simulink model "Fahrdynamikregelung"  (R2022b)
settings: Solver=ode1  StartTime=0.0  StopTime=10.0  FixedStep=Ts  RelTol=1e-3
InitFcn:
  | run("Fzg_Par.m")
values from neighbouring files (symbols this model uses):
  aero_balance_rear = 55/100    (= 0.55)    [Fzg_Par.m]    (also in Fzg_par.m)
  c_alpha_H = 13400    [Fzg_Par.m]    (also in Fzg_par.m)
  c_alpha_V = 9300    [Fzg_Par.m]    (also in Fzg_par.m)
  c_DA = 3.9    [Fzg_Par.m]    (also in Fzg_par.m)
  Dyn_Reifenradius = 0.23    [Fzg_Par.m]    (also in Fzg_par.m)
  h_COG = 300/1000    (= 0.3)    [Fzg_Par.m]    (also in Fzg_par.m)
  J_Rad = 0.2656    [Fzg_Par.m]
  K_PD = 5    [Fzg_Par.m]
  K_T = 0.62    [Fzg_Par.m]
  L001_APPS1 = [7.99989318848 7.99989318848 7.99989318848 7.99989318848 7.99989318848 7.99989318848 7.99989318848 7.99989318848 7.99989318848 7.99989318848 7.99989318848 7.99989318848 ... (3961 elements, 3961x1)]    [TestData24.mat]
  L001_GPSSpeed = [0.148407205939 0.148407205939 0.148407205939 0.148407205939 0.148407205939 0.148407205939 0.148407205939 0.148407205939 0.148407205939 0.148407205939 0.153283953667 0.202051386237 ... (3961 elements, 3961x1)]    [TestData24.mat]
  L001_InlineAcc = [-0.0102365128696 -0.0101919434965 -0.00925597175956 -0.0068023907952 -0.00259832036681 0.00465657003224 0.0166592858732 0.0341619476676 0.0555711686611 0.0739719197154 0.0942579805851 0.102946907282 ... (3961 elements, 3961x1)]    [TestData24.mat]
  L001_INVRERPM = [228.575454712 228.575454712 228.575454712 228.575454712 228.575454712 228.575454712 228.575454712 228.575454712 228.575454712 228.575454712 229.405059814 237.701187134 ... (3961 elements, 3961x1)]    [TestData24.mat]
  L001_LateralAcc = [-0.171782910824 -0.171881780028 -0.171881780028 -0.171881780028 -0.17187024653 -0.171626374125 -0.171095818281 -0.169845193624 -0.168227121234 -0.169884741306 -0.173443824053 -0.169364064932 ... (3961 elements, 3961x1)]    [TestData24.mat]
  L001_Steeringangle = [-0.000259418739006 -0.000259418739006 -0.000259418739006 -0.000259418739006 -0.000259418739006 -0.000259418739006 -0.000259418739006 -0.000259418739006 -0.000259418739006 -0.000259418739006 -0.000259418739006 -0.000259418739006 ... (3961 elements, 3961x1)]    [TestData24.mat]
  L001_time = [0 0.019999999553 0.0399999991059 0.0599999986589 0.0799999982119 0.10000000149 0.119999997318 0.140000000596 0.159999996424 0.180000007153 0.20000000298 0.219999998808 ... (3961 elements, 3961x1)]    [TestData24.mat]
  L001_YawRate = [0.023690149188 0.0136420829222 0.00359401665628 -0.0035233637318 -0.0120642203838 -0.0241218991578 -0.0424596183002 -0.0578666552901 -0.0431294925511 0.0049337586388 0.0141444858164 -0.0101383412257 ... (3961 elements, 3961x1)]    [TestData24.mat]
  L038_ACcurrentINVL = [99.4390869141 109.504394531 119.569709778 129.252166748 135.488876343 141.725585938 147.962295532 154.199005127 160.137954712 163.397140503 166.656311035 169.915481567 ... (1550 elements, 1550x1)]    [Lap38Data.mat]
  L038_ACcurrentINVR = [20.6730155945 25.7066345215 30.7402534485 36.3266334534 46.8878517151 57.4490699768 68.0102920532 78.5715103149 88.6779708862 94.6916427612 100.705307007 106.718971252 ... (1550 elements, 1550x1)]    [Lap38Data.mat]
  L038_DCcurrentINVL = [23.7739772797 26.0139312744 28.2538833618 30.4728279114 32.5027122498 34.5325965881 36.5624809265 38.5923652649 40.5376625061 41.7216491699 42.9056396484 44.089630127 ... (1550 elements, 1550x1)]    [Lap38Data.mat]
  L038_DCcurrentINVR = [4.40954971313 5.53267717361 6.65580463409 7.92606782913 10.5205507278 13.1150331497 15.7095165253 18.3039989471 20.8878383636 23.3758850098 25.8639297485 28.3519744873 ... (1550 elements, 1550x1)]    [Lap38Data.mat]
  L038_time = [0 0.019999999553 0.0399999991059 0.0599999986589 0.0799999982119 0.10000000149 0.119999997318 0.140000000596 0.159999996424 0.180000007153 0.20000000298 0.219999998808 ... (1550 elements, 1550x1)]    [Lap38Data.mat]    (also in Testrunde_PATZE.mat)
  L038_VTS = [491.347839355 491.925415039 492.502990723 492.660247803 489.034515381 485.408782959 481.783050537 478.157287598 474.759063721 473.408447266 472.057830811 470.707214355 ... (1550 elements, 1550x1)]    [Lap38Data.mat]
  l_fzg = 1300/1000    (= 1.3)    [Fzg_Par.m]    (also in Fzg_par.m)
  l_H_fzg = 507/1000    (= 0.507)    [Fzg_Par.m]    (also in Fzg_par.m)
  l_V_fzg = 1023/1000    (= 1.023)    [Fzg_Par.m]    (also in Fzg_par.m)
  m_Front = m_fzg * 0.4    (= 129.4)    [Fzg_Par.m]    (also in Fzg_par.m)
  m_fzg = 241.5 + 82    (= 323.5)    [Fzg_Par.m]    (also in Fzg_par.m)
  m_Rear = m_fzg - m_Front    (= 194.1)    [Fzg_Par.m]    (also in Fzg_par.m)
  ss_A = [-(c_alpha_V*l_V_fzg^2+c_alpha_H*l_H_fzg^2)/(J_fzg_z*v_x) (c_alpha_H*l_H_fzg-c_alpha_V*l_V_fzg)/J_fzg_z ... (first row only)    [Fzg_Par.m]    (also in Fzg_par.m)
  ss_B = [(c_alpha_V*l_V_fzg)/J_fzg_z -(c_alpha_H*l_H_fzg)/J_fzg_z ... (first row only)    [Fzg_Par.m]    (also in Fzg_par.m)
  ss_C = [1 0]    [Fzg_Par.m]    (also in Fzg_par.m)
  ss_D = [0 0]    [Fzg_Par.m]    (also in Fzg_par.m)
  t_H_fzg = 1200/1000    (= 1.2)    [Fzg_Par.m]    (also in Fzg_par.m)
  T_p = T_v/10    (= 0.01)    [Fzg_Par.m]
  T_v = 0.1    [Fzg_Par.m]
libraries: simulink x2
settings Model: Creator=timos  LastModifiedBy=timos

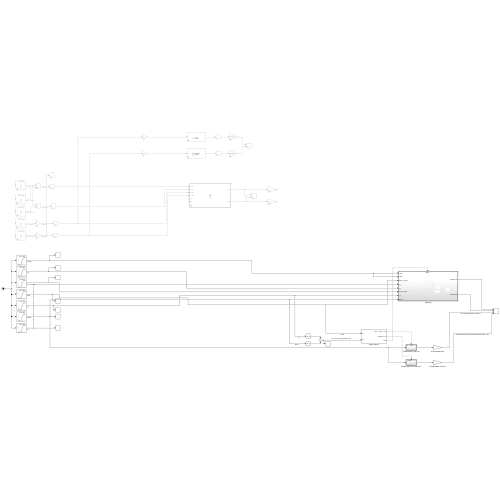
[thumbnail: Simulink's stored preview of the top-level diagram]
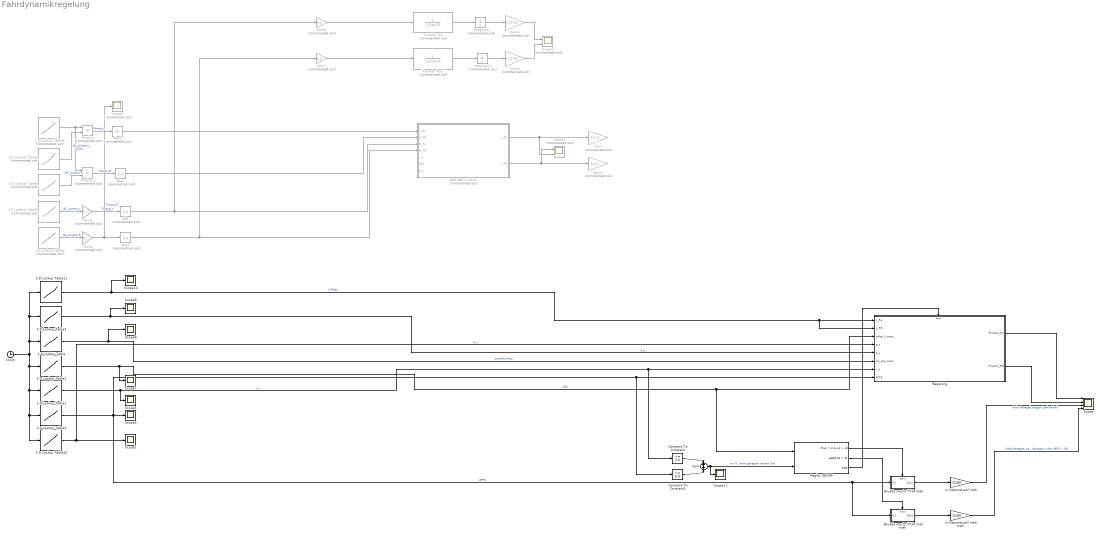
== system Fahrdynamikregelung ==
  1-D Lookup Table : Lookup_n-D  NumberOfTableDimensions=1  BreakpointsForDimension1=L001_time  Table=L001_YawRate  InternalRulePriority=Speed  RndMeth=Simplest
  1-D Lookup Table1 : Lookup_n-D  NumberOfTableDimensions=1  BreakpointsForDimension1=L001_time  Table=L001_GPSSpeed/3.6  InternalRulePriority=Speed  RndMeth=Simplest
  1-D Lookup Table10 : Lookup_n-D  NumberOfTableDimensions=1  BreakpointsForDimension1=L001_time  Table=L001_InlineAcc*9.81  InternalRulePriority=Speed  RndMeth=Simplest
  1-D Lookup Table11 : Lookup_n-D  NumberOfTableDimensions=1  BreakpointsForDimension1=L001_time  Table=L001_INVRERPM/(10*60*4.3)  InternalRulePriority=Speed  RndMeth=Simplest
  1-D Lookup Table2 : Lookup_n-D  NumberOfTableDimensions=1  BreakpointsForDimension1=L001_time  Table=L001_Steeringangle*0.36  InternalRulePriority=Speed  RndMeth=Simplest
  1-D Lookup Table3 : Lookup_n-D  NumberOfTableDimensions=1  BreakpointsForDimension1=L001_time  Table=L001_LateralAcc*9.81  InternalRulePriority=Speed  RndMeth=Simplest
  1-D Lookup Table4 : Lookup_n-D  NumberOfTableDimensions=1  BreakpointsForDimension1=L001_time  Table=L001_APPS1  InternalRulePriority=Speed  RndMeth=Simplest
  1-D Lookup Table5 : Lookup_n-D  Commented=on  NumberOfTableDimensions=1  BreakpointsForDimension1=L038_time  Table=L038_DCcurrentINVL  InternalRulePriority=Speed  RndMeth=Simplest
  1-D Lookup Table6 : Lookup_n-D  Commented=on  NumberOfTableDimensions=1  BreakpointsForDimension1=L038_time  Table=L038_DCcurrentINVR  InternalRulePriority=Speed  RndMeth=Simplest
  1-D Lookup Table7 : Lookup_n-D  Commented=on  NumberOfTableDimensions=1  BreakpointsForDimension1=L038_time  Table=L038_ACcurrentINVL  InternalRulePriority=Speed  RndMeth=Simplest
  1-D Lookup Table8 : Lookup_n-D  Commented=on  NumberOfTableDimensions=1  BreakpointsForDimension1=L038_time  Table=L038_ACcurrentINVR  InternalRulePriority=Speed  RndMeth=Simplest
  1-D Lookup Table9 : Lookup_n-D  Commented=on  NumberOfTableDimensions=1  BreakpointsForDimension1=L038_time  Table=L038_VTS  InternalRulePriority=Speed  RndMeth=Simplest
  Abs{,1..3} (4 alike) : Abs  Commented=on  SaturateOnIntegerOverflow=off
  Brudda macht TY24 meh : Subsystem  TreatAsAtomicUnit=on
  Brudda macht TY24 meh meh : Subsystem  TreatAsAtomicUnit=on
  Clock : Clock
  Compare To Constant : simulink/Logic and Bit Operations/Compare To Constant  relop=<=  const=2.0  OutDataTypeStr=boolean
  Compare To Constant1 : simulink/Logic and Bit Operations/Compare To Constant  relop=<=  const=5.0  OutDataTypeStr=boolean
  Gain : Gain  Commented=on  Gain=1/4.3
  Gain1 : Gain  Commented=on  Gain=K_T
  Gain2 : Gain  Commented=on  Gain=K_T
  Gain3 : Gain  Commented=on  Gain=1/4.3
  Gain4 : Gain  Commented=on  Gain=1/(2*pi)
  Gain5 : Gain  Commented=on  Gain=1/(2*pi)
  Gain6 : Gain  Commented=on  Gain=4.3
  Gain7 : Gain  Commented=on  Gain=4.3
  Integrator : Integrator  Commented=on
  Integrator1 : Integrator  Commented=on
  MATLAB Function : MATLAB Function  Commented=on  TreatAsAtomicUnit=on
  Product : Product  Commented=on
  Product1 : Product  Commented=on
  Regelung : Subsystem
  Regler ON/OFF : If  NumInputs=2  IfExpression=u1 < 3 & u1 > -3  ElseIfExpressions=u2 > 0
  Scope : Scope  NumInputPorts=4
  Scope{1,4..5,7..11} (8 alike) : Scope
  Scope2 : Scope  Commented=on  NumInputPorts=2
  Scope3 : Scope  Commented=on  NumInputPorts=2
  Scope6 : Scope  Commented=on
  Sum : Sum  Inputs=+|+  OutDataTypeStr=double
  Transfer Fcn : TransferFcn  Commented=on  Denominator=[J_Rad 0]
  Transfer Fcn1 : TransferFcn  Commented=on  Denominator=[J_Rad 0]
  in Dezimalzahl meh : Gain  Gain=1/100
  in Dezimalzahl meh meh : Gain  Gain=1/100
  wires:
  Clock/1 -> 1-D Lookup Table/1, 1-D Lookup Table11/1, 1-D Lookup Table3/1, 1-D Lookup Table2/1, 1-D Lookup Table10/1, 1-D Lookup Table4/1, 1-D Lookup Table1/1
  1-D Lookup Table3/1 -> Scope9/1, Regelung/5(a_y)  "a_y"
  1-D Lookup Table5/1 -> Product/2  "DC_current_L"
  1-D Lookup Table7/1 -> Gain2/1  "AC_current_L"
  1-D Lookup Table8/1 -> Gain1/1  "AC_current_R"
  Gain2/1 -> Abs/1  "Torque_L"
  Gain1/1 -> Abs1/1, Scope6/1  "Torque_R"
  1-D Lookup Table9/1 -> Product1/1, Product/1  "V_TS"
  1-D Lookup Table6/1 -> Product1/2  "DC_current_R"
  Product/1 -> Abs3/1  "Power_L"
  Product1/1 -> Abs2/1  "Power_R"
  Abs/1 -> Gain6/1, MATLAB Function/3(M_RL)
  Abs1/1 -> Gain7/1, MATLAB Function/4(M_RR)
  Abs2/1 -> MATLAB Function/2(P_RR)
  Abs3/1 -> MATLAB Function/1(P_RL)
  MATLAB Function/1(n_RL) -> Scope2/2, Gain/1
  MATLAB Function/2(n_RR) -> Scope2/1, Gain3/1
  1-D Lookup Table/1 -> Scope8/1, Regelung/6(psi_dot_mess)  "psi_dot_mess"
  1-D Lookup Table4/1 -> Regelung/8(APPS), Compare To Constant1/1, Scope4/1, Brudda macht TY24 meh meh/1(In1), Brudda macht TY24 meh/1(In1)  "APPS"
  1-D Lookup Table1/1 -> Scope5/1, Regelung/7(v_x), Compare To Constant/1  "v_x"
  1-D Lookup Table2/1 -> Scope7/1, Regler ON/OFF/1, Regelung/3("delta_V_mess ")  "SAS"
  1-D Lookup Table10/1 -> Scope1/1, Regelung/4(a_x)  "a_x"
  Regelung/2(Produkt_RR) -> Scope/2
  Regelung/1(Produkt_RL) -> Scope/1
  Brudda macht TY24 meh/1(Out1) -> in Dezimalzahl meh/1
  Transfer Fcn1/1 -> Integrator1/1
  Transfer Fcn/1 -> Integrator/1
  Integrator1/1 -> Gain5/1
  Integrator/1 -> Gain4/1
  Gain4/1 -> Scope3/1
  Gain5/1 -> Scope3/2
  Gain7/1 -> Transfer Fcn1/1
  Gain6/1 -> Transfer Fcn/1
  1-D Lookup Table11/1 -> Scope10/1, Regelung/2(n_RR), Regelung/1(n_RL)  "n_Rear"
  in Dezimalzahl meh/1 -> Scope/3  "Nicht Geregelt wegen Lenkwinkel"
  in Dezimalzahl meh meh/1 -> Scope/4  "Nicht Geregelt wegen Arschlangsam oder APPS < 5%"
  Brudda macht TY24 meh meh/1(Out1) -> in Dezimalzahl meh meh/1
  Regler ON/OFF/1 -> Brudda macht TY24 meh/Action
  Regler ON/OFF/2 -> Brudda macht TY24 meh meh/Action
  Regler ON/OFF/3 -> Regelung/Action
  Compare To Constant/1 -> Sum/1
  Compare To Constant1/1 -> Sum/2
  Sum/1 -> Scope11/1, Regler ON/OFF/2  "nur 0, wenn geregelt werden Soll"

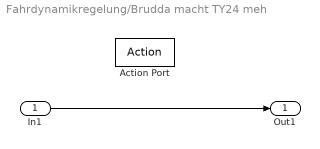
== system Fahrdynamikregelung/Brudda macht TY24 meh ==
  In1 : Inport
  Action Port : ActionPort  ActionPortLabel=if(u1 < 3 & u1 > -3)
  Out1 : Outport
  wires:
  In1/1 -> Out1/1

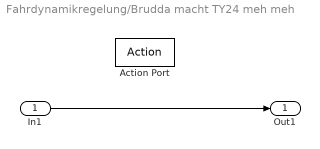
== system Fahrdynamikregelung/Brudda macht TY24 meh meh ==
  In1 : Inport
  Action Port : ActionPort  ActionPortLabel=elseif(u2 > 0)
  Out1 : Outport
  wires:
  In1/1 -> Out1/1

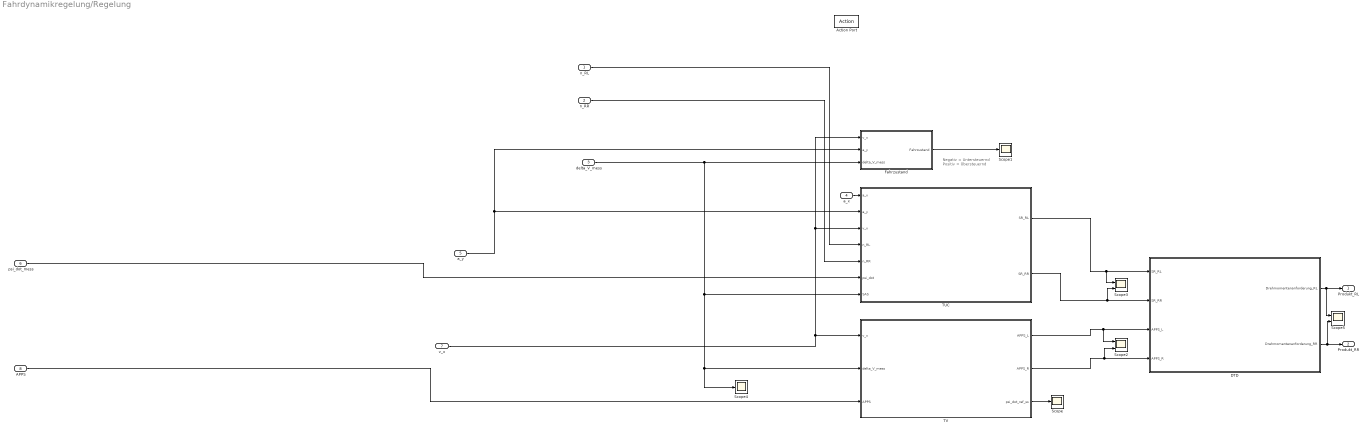
== system Fahrdynamikregelung/Regelung ==
  note: Negativ = Untersteuernd
      | Positiv = Übersteuernd
  n_RL : Inport
  n_RR : Inport  Port=2
  "delta_V_mess " : Inport  Port=3
  a_x : Inport  Port=4
  a_y : Inport  Port=5
  psi_dot_mess : Inport  Port=6
  v_x : Inport  Port=7
  APPS : Inport  Port=8
  Action Port : ActionPort  ActionPortLabel=else
  DTD : Subsystem
  Fahrzustand : Subsystem
  Scope : Scope
  Scope1 : Scope
  Scope2 : Scope  NumInputPorts=2
  Scope3 : Scope  NumInputPorts=2
  Scope4 : Scope
  Scope5 : Scope  NumInputPorts=2
  TUC : Subsystem
  TV : Subsystem
  Produkt_RL : Outport
  Produkt_RR : Outport  Port=2
  wires:
  v_x/1 -> Fahrzustand/1(v_x), TUC/3(v_x), TV/1(v_x)
  a_y/1 -> TUC/2(a_y), Fahrzustand/2(a_y)
  n_RR/1 -> TUC/5(n_RR)
  TUC/1(SR_RL) -> Scope3/1, DTD/1(SR_RL)
  TUC/2(SR_RR) -> Scope3/2, DTD/2(SR_RR)
  Fahrzustand/1(Fahrzustand) -> Scope1/1
  TV/1(APPS_L) -> Scope2/1, DTD/3(APPS_L)
  TV/3(psi_dot_ref_ss) -> Scope/1
  TV/2(APPS_R) -> Scope2/2, DTD/4(APPS_R)
  psi_dot_mess/1 -> TUC/6(psi_dot)
  n_RL/1 -> TUC/4(n_RL)
  APPS/1 -> TV/3(APPS)
  a_x/1 -> TUC/1(a_x)
  "delta_V_mess "/1 -> TV/2(delta_V_mess), Scope4/1, TUC/7(SAS), Fahrzustand/3("delta_V_mess ")
  DTD/1(Drehmomentenanforderung_RL) -> Scope5/1, Produkt_RL/1
  DTD/2(Drehmomentenanforderung_RR) -> Scope5/2, Produkt_RR/1

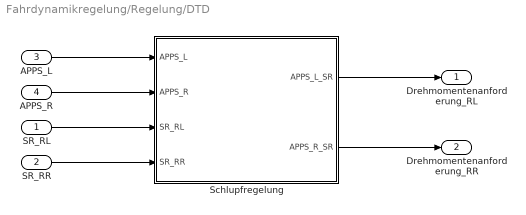
== system Fahrdynamikregelung/Regelung/DTD ==
  SR_RL : Inport
  SR_RR : Inport  Port=2
  APPS_L : Inport  Port=3
  APPS_R : Inport  Port=4
  Schlupfregelung : MATLAB Function  TreatAsAtomicUnit=on
  Drehmomentenanforderung_RL : Outport
  Drehmomentenanforderung_RR : Outport  Port=2
  wires:
  APPS_L/1 -> Schlupfregelung/1(APPS_L)
  Schlupfregelung/2(APPS_R_SR) -> Drehmomentenanforderung_RR/1
  Schlupfregelung/1(APPS_L_SR) -> Drehmomentenanforderung_RL/1
  SR_RL/1 -> Schlupfregelung/3(SR_RL)
  APPS_R/1 -> Schlupfregelung/2(APPS_R)
  SR_RR/1 -> Schlupfregelung/4(SR_RR)

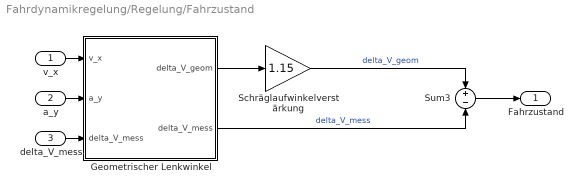
== system Fahrdynamikregelung/Regelung/Fahrzustand ==
  v_x : Inport
  a_y : Inport  Port=2
  "delta_V_mess " : Inport  Port=3
  Geometrischer Lenkwinkel : MATLAB Function  TreatAsAtomicUnit=on
  Schräglaufwinkelverstärkung : Gain  Gain=1.15
  Sum3 : Sum  Inputs=+|-
  Fahrzustand : Outport
  wires:
  Geometrischer Lenkwinkel/1(delta_V_geom) -> Schräglaufwinkelverstärkung/1
  Geometrischer Lenkwinkel/2(delta_V_mess) -> Sum3/2  "delta_V_mess"
  Schräglaufwinkelverstärkung/1 -> Sum3/1  "delta_V_geom"
  v_x/1 -> Geometrischer Lenkwinkel/1(v_x)
  a_y/1 -> Geometrischer Lenkwinkel/2(a_y)
  "delta_V_mess "/1 -> Geometrischer Lenkwinkel/3("delta_V_mess ")
  Sum3/1 -> Fahrzustand/1

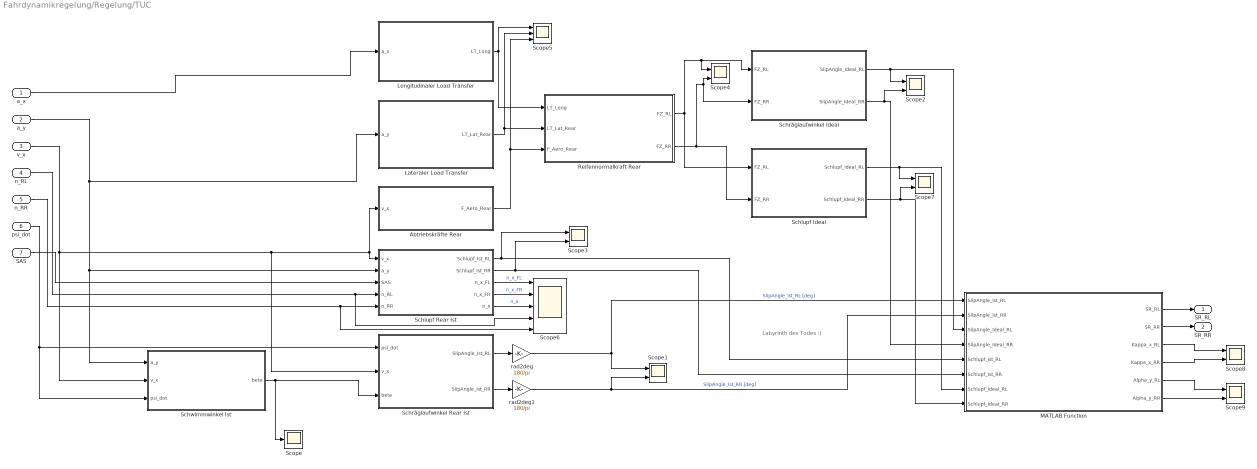
== system Fahrdynamikregelung/Regelung/TUC ==
  note: Labyrinth des Todes :)
  a_x : Inport
  a_y : Inport  Port=2
  v_x : Inport  Port=3
  n_RL : Inport  Port=4
  n_RR : Inport  Port=5
  psi_dot : Inport  Port=6
  SAS : Inport  Port=7
  Abtriebskräfte Rear : MATLAB Function  TreatAsAtomicUnit=on
  Lateraler Load Transfer : MATLAB Function  TreatAsAtomicUnit=on
  Longitudinaler Load Transfer : MATLAB Function  TreatAsAtomicUnit=on
  MATLAB Function : MATLAB Function  TreatAsAtomicUnit=on
  Reifennormalkraft Rear : MATLAB Function  TreatAsAtomicUnit=on
  Schlupf Ideal : MATLAB Function  TreatAsAtomicUnit=on
  Schlupf Rear Ist : MATLAB Function  TreatAsAtomicUnit=on
  Schräglaufwinkel Ideal : MATLAB Function  TreatAsAtomicUnit=on
  Schräglaufwinkel Rear Ist : MATLAB Function  TreatAsAtomicUnit=on
  Schwimmwinkel Ist : Subsystem
  Scope : Scope
  Scope{1..4,7..9} (7 alike) : Scope  NumInputPorts=2
  Scope5 : Scope  NumInputPorts=3
  Scope6 : Scope  NumInputPorts=5
  rad2deg : Gain  Gain=180/pi
  rad2deg1 : Gain  Gain=180/pi
  SR_RL : Outport
  SR_RR : Outport  Port=2
  wires:
  Lateraler Load Transfer/1(LT_Lat_Rear) -> Scope5/2, Reifennormalkraft Rear/2(LT_Lat_Rear)
  Abtriebskräfte Rear/1(F_Aero_Rear) -> Scope5/3, Reifennormalkraft Rear/3(F_Aero_Rear)
  Schlupf Rear Ist/2(Schlupf_Ist_RR) -> Scope3/2, MATLAB Function/6(Schlupf_Ist_RR)
  Longitudinaler Load Transfer/1(LT_Long) -> Scope5/1, Reifennormalkraft Rear/1(LT_Long)
  Schwimmwinkel Ist/1(beta) -> Scope/1, Schräglaufwinkel Rear Ist/3(beta)
  Reifennormalkraft Rear/1(FZ_RL) -> Schlupf Ideal/1(FZ_RL), Scope4/1, Schräglaufwinkel Ideal/1(FZ_RL)
  Schlupf Ideal/1(Schlupf_Ideal_RL) -> Scope7/1, MATLAB Function/7(Schlupf_Ideal_RL)
  Schräglaufwinkel Ideal/1(SlipAngle_Ideal_RL) -> Scope2/1, MATLAB Function/3(SlipAngle_Ideal_RL)
  Schräglaufwinkel Rear Ist/2(SlipAngle_Ist_RR) -> rad2deg1/1
  Schlupf Rear Ist/1(Schlupf_Ist_RL) -> Scope3/1, MATLAB Function/5(Schlupf_Ist_RL)
  Schräglaufwinkel Ideal/2(SlipAngle_Ideal_RR) -> Scope2/2, MATLAB Function/4(SlipAngle_Ideal_RR)
  Reifennormalkraft Rear/2(FZ_RR) -> Schlupf Ideal/2(FZ_RR), Scope4/2, Schräglaufwinkel Ideal/2(FZ_RR)
  Schlupf Ideal/2(Schlupf_Ideal_RR) -> Scope7/2, MATLAB Function/8(Schlupf_Ideal_RR)
  Schräglaufwinkel Rear Ist/1(SlipAngle_Ist_RL) -> rad2deg/1
  MATLAB Function/1(SR_RL) -> SR_RL/1
  MATLAB Function/2(SR_RR) -> SR_RR/1
  a_y/1 -> Lateraler Load Transfer/1(a_y), Schwimmwinkel Ist/1(a_y), Schlupf Rear Ist/2(a_y)
  v_x/1 -> Abtriebskräfte Rear/1(v_x), Schlupf Rear Ist/1(v_x), Schräglaufwinkel Rear Ist/2(v_x), Schwimmwinkel Ist/2(v_x)
  n_RL/1 -> Scope6/4, Schlupf Rear Ist/4(n_RL)
  n_RR/1 -> Scope6/5, Schlupf Rear Ist/5(n_RR)
  psi_dot/1 -> Schwimmwinkel Ist/3(psi_dot), Schräglaufwinkel Rear Ist/1(psi_dot)
  a_x/1 -> Longitudinaler Load Transfer/1(a_x)
  rad2deg/1 -> Scope1/1, MATLAB Function/1(SlipAngle_Ist_RL)  "SlipAngle_Ist_RL [deg]"
  rad2deg1/1 -> Scope1/2, MATLAB Function/2(SlipAngle_Ist_RR)  "SlipAngle_Ist_RR [deg]"
  SAS/1 -> Schlupf Rear Ist/3(SAS)
  Schlupf Rear Ist/4(n_x_FR) -> Scope6/2  "n_x_FR"
  Schlupf Rear Ist/3(n_x_FL) -> Scope6/1  "n_x_FL"
  Schlupf Rear Ist/5(n_x) -> Scope6/3  "n_x"
  MATLAB Function/3(Kappa_x_RL) -> Scope8/1
  MATLAB Function/4(Kappa_x_RR) -> Scope8/2
  MATLAB Function/6(Alpha_y_RR) -> Scope9/2
  MATLAB Function/5(Alpha_y_RL) -> Scope9/1

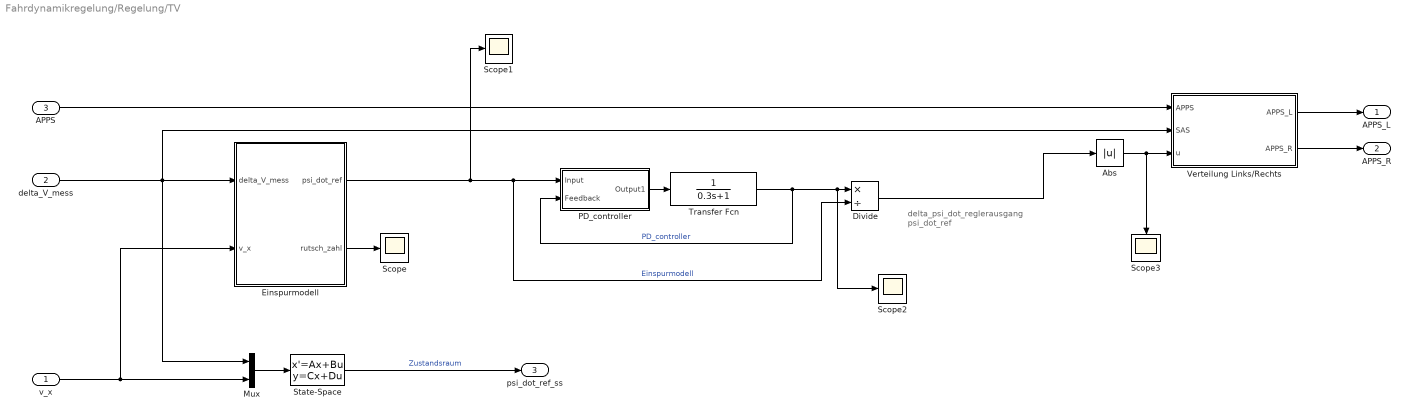
== system Fahrdynamikregelung/Regelung/TV ==
  note: delta_psi_dot_reglerausgang
      | psi_dot_ref
  v_x : Inport
  delta_V_mess : Inport  Port=2
  APPS : Inport  Port=3
  Abs : Abs  SaturateOnIntegerOverflow=off
  Divide : Product  Inputs=*/
  Einspurmodell : MATLAB Function  TreatAsAtomicUnit=on
  Mux : Mux  Inputs=2
  PD_controller : Subsystem
  Scope{,1..3} (4 alike) : Scope
  State-Space : StateSpace  A=ss_A  B=ss_B  C=ss_C  D=ss_D  InitialCondition=0
  Transfer Fcn : TransferFcn  Denominator=[0.3 1]
  Verteilung Links/Rechts : MATLAB Function  TreatAsAtomicUnit=on
  APPS_L : Outport
  APPS_R : Outport  Port=2
  psi_dot_ref_ss : Outport  Port=3
  wires:
  Mux/1 -> State-Space/1
  Einspurmodell/1(psi_dot_ref) -> Scope1/1, Divide/2, PD_controller/1(Input)  "Einspurmodell"
  v_x/1 -> Einspurmodell/2(v_x), Mux/2
  Einspurmodell/2(rutsch_zahl) -> Scope/1
  delta_V_mess/1 -> Verteilung Links/Rechts/2(SAS), Einspurmodell/1(delta_V_mess), Mux/1
  State-Space/1 -> psi_dot_ref_ss/1  "Zustandsraum"
  PD_controller/1(Output1) -> Transfer Fcn/1
  Transfer Fcn/1 -> Scope2/1, Divide/1, PD_controller/2(Feedback)  "PD_controller"
  Divide/1 -> Abs/1
  APPS/1 -> Verteilung Links/Rechts/1(APPS)
  Verteilung Links/Rechts/2(APPS_R) -> APPS_R/1
  Verteilung Links/Rechts/1(APPS_L) -> APPS_L/1
  Abs/1 -> Verteilung Links/Rechts/3(u), Scope3/1

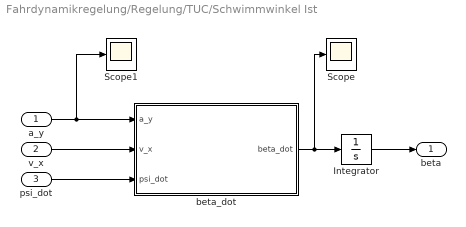
== system Fahrdynamikregelung/Regelung/TUC/Schwimmwinkel Ist ==
  a_y : Inport
  v_x : Inport  Port=2
  psi_dot : Inport  Port=3
  Integrator : Integrator
  Scope : Scope
  Scope1 : Scope
  beta_dot : MATLAB Function  TreatAsAtomicUnit=on
  beta : Outport
  wires:
  v_x/1 -> beta_dot/2(v_x)
  a_y/1 -> Scope1/1, beta_dot/1(a_y)
  psi_dot/1 -> beta_dot/3(psi_dot)
  beta_dot/1(beta_dot) -> Scope/1, Integrator/1
  Integrator/1 -> beta/1

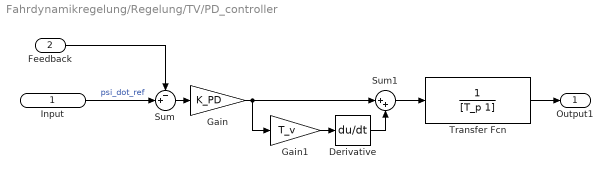
== system Fahrdynamikregelung/Regelung/TV/PD_controller ==
  Input : Inport
  Feedback : Inport  Port=2
  Derivative : Derivative
  Gain : Gain  Gain=K_PD
  Gain1 : Gain  Gain=T_v
  Sum : Sum  Inputs=-+|
  Sum1 : Sum  Inputs=|++
  Transfer Fcn : TransferFcn  Denominator=[T_p 1]
  Output1 : Outport
  wires:
  Feedback/1 -> Sum/1
  Gain1/1 -> Derivative/1
  Sum1/1 -> Transfer Fcn/1
  Gain/1 -> Gain1/1, Sum1/1
  Input/1 -> Sum/2  "psi_dot_ref"
  Sum/1 -> Gain/1
  Derivative/1 -> Sum1/2
  Transfer Fcn/1 -> Output1/1

== matlab function Fahrdynamikregelung/Regelung/TUC/Schräglaufwinkel Rear Ist ==
  data: psi_dot input; SlipAngle_Ist_RL output; SlipAngle_Ist_RR output; v_x input; beta input; l_H_fzg parameter
function [SlipAngle_Ist_RL,SlipAngle_Ist_RR] = fcn(psi_dot,v_x,beta,l_H_fzg)

    SlipAngle_Ist_RL = (deg2rad(psi_dot)*l_H_fzg/v_x) + deg2rad(beta);
    SlipAngle_Ist_RR = SlipAngle_Ist_RL;

== matlab function Fahrdynamikregelung/Regelung/TUC/Schwimmwinkel Ist/beta_dot ==
  data: a_y input; beta_dot output; v_x input; psi_dot input
function beta_dot  = Schwimmwinkel(a_y,v_x,psi_dot)

    beta_dot = (a_y/v_x) - deg2rad(psi_dot);

== matlab function Fahrdynamikregelung/Regelung/TUC/Schräglaufwinkel Ideal ==
  data: FZ_RL input; SlipAngle_Ideal_RL output; FZ_RR input; SlipAngle_Ideal_RR output; Sturzwinkel parameter
function [SlipAngle_Ideal_RL,SlipAngle_Ideal_RR] = SlipAngle_Ideal(FZ_RL,FZ_RR,Sturzwinkel)
% Scaling und Shape Koeffizienten
FZ0                 = +8.000e+002;
LFZO  				= 1;
LCY   				= 0.90;
LMUY  				= 0.75;
LEY   				= 1;
LKY   				= 1;
LHY   				= 0;
LVY   				= 0;
LGAY  				= 0.75;
% Laterale Koeffizienten
PCY1				= +1.625E+000;
PDY1				= +2.554E+000;
PDY2				= -4.021E-001;
PDY3				= +5.406E+000;
PEY1				= +1.715E-001;
PEY2				= -8.339E-001;
PEY3				= -1.743E-001;
PEY4				= -6.110E+000;
PKY1				= -5.912E+001;
PKY2				= +2.567E+000;
PKY3				= +4.787E-001;
PHY1				= +0.000E+000;
PHY2				= +0.000E+000;
PHY3				= -2.152E-002;
PVY1				= +0.000E+000;
PVY2				= +0.000E+000;
PVY3				= -2.151E+000;
PVY4				= -8.772E-001;
% =======================================================================
% RL
i = 0;
Fz = FZ_RL;
GAMMA = Sturzwinkel;
FY_RL = zeros((12/0.1+1),3);                                                  % Vorinitialisierung
for ALPHA = 0:0.1:12
    % ====================================================================
    % Magic Formula Berechnung FX // Nur Längsschlupf
    ALPHA  =  ALPHA.*pi/180;
    GAMMA  =  GAMMA.*pi/180;
    FZ0PR  = FZ0  .*  LFZO;
    DFZ    = (Fz - FZ0PR) ./ FZ0PR;

    GAMMAY = GAMMA .* LGAY;
    SHY = (PHY1 + PHY2 .* DFZ) .* LHY + PHY3 .* GAMMAY;
    ALPHAY = ALPHA + SHY;
    CY = PCY1 .* LCY;
    MUY = (PDY1 + PDY2 .* DFZ) .* (1 - PDY3 .* GAMMAY.^2) .* LMUY;
    DY = MUY .* Fz;
    EY = (PEY1 + PEY2 .* DFZ) .* (1 - (PEY3 + PEY4 .* GAMMAY) .* sign(ALPHAY)) .* LEY;
    KY = PKY1 .* FZ0 .* sin(2 * atan(Fz ./ (PKY2 .* FZ0 .* LFZO))) .* (1 - PKY3 .* abs(GAMMAY)) .* LFZO .* LKY;
    BY = KY ./ (CY .* DY);
    SVY = Fz .* ((PVY1 + PVY2 .* DFZ) .* LVY + (PVY3 + PVY4 .* DFZ) .* GAMMAY) .* LMUY;
    % ====================================================================
    % Eintragung in die Matrix
    i=i+1;
    FY_RL(i,1) = Fz;
    FY_RL(i,2) = rad2deg(ALPHA);
    FY_RL(i,3) = abs(DY .* sin(CY .* atan(BY .* ALPHAY - EY .* (BY .* ALPHAY - atan(BY .* ALPHAY)))) + SVY);
end
[~, Index] = max(FY_RL(:,3));                                               % Zeilennummer des maximalen FX-Werte
SlipAngle_Ideal_RL = FY_RL(Index,2);                                        % Eintragung in die Ausgabegröße
% =======================================================================
% RR
i = 0;
Fz = FZ_RR;
GAMMA = Sturzwinkel;
FY_RR = zeros((12/0.1+1),3);                                                  % Vorinitialisierung
for ALPHA = 0:0.1:12
    % ====================================================================
    % Magic Formula Berechnung FX // Nur Längsschlupf
    ALPHA  =  ALPHA.*pi/180;
    GAMMA  =  GAMMA.*pi/180;
    FZ0PR  = FZ0  .*  LFZO;
    DFZ    = (Fz - FZ0PR) ./ FZ0PR;
    GAMMAY = GAMMA .* LGAY;
    SHY = (PHY1 + PHY2 .* DFZ) .* LHY + PHY3 .* GAMMAY;
    ALPHAY = ALPHA + SHY;
    CY = PCY1 .* LCY;
    MUY = (PDY1 + PDY2 .* DFZ) .* (1 - PDY3 .* GAMMAY.^2) .* LMUY;
    DY = MUY .* Fz;
    EY = (PEY1 + PEY2 .* DFZ) .* (1 - (PEY3 + PEY4 .* GAMMAY) .* sign(ALPHAY)) .* LEY;
    KY = PKY1 .* FZ0 .* sin(2 * atan(Fz ./ (PKY2 .* FZ0 .* LFZO))) .* (1 - PKY3 .* abs(GAMMAY)) .* LFZO .* LKY;
    BY = KY ./ (CY .* DY);
    SVY = Fz .* ((PVY1 + PVY2 .* DFZ) .* LVY + (PVY3 + PVY4 .* DFZ) .* GAMMAY) .* LMUY;
    % ====================================================================
    % Eintragung in die Matrix
    i=i+1;
    FY_RR(i,1) = Fz;
    FY_RR(i,2) = rad2deg(ALPHA);
    FY_RR(i,3) = abs(DY .* sin(CY .* atan(BY .* ALPHAY - EY .* (BY .* ALPHAY - atan(BY .* ALPHAY)))) + SVY);
end
[~, Index] = max(FY_RR(:,3));                                               % Zeilennummer des maximalen FX-Werte
SlipAngle_Ideal_RR = FY_RR(Index,2);                                        % Eintragung in die Ausgabegröße

== matlab function Fahrdynamikregelung/Regelung/TUC/Schlupf Ideal ==
  data: FZ_RL input; Schlupf_Ideal_RL output; FZ_RR input; Schlupf_Ideal_RR output; Sturzwinkel parameter
function [Schlupf_Ideal_RL,Schlupf_Ideal_RR] = Schlupf_Ideal(FZ_RL,FZ_RR,Sturzwinkel)
% =======================================================================
% Magic Formula Parameter
FZ0                 = +8.000e+002;
LFZO  				= 1;
% Scaling und Shape Koeffizienten
LCX   				= 1;
LMUX  				= 0.75;
LEX   				= 1;
LKX   				= 1;
LHX   				= 1;
LVX   				= 1;
LGAX  				= 1;
% Longitudinal Koeffizienten
PCX1  				= +1.786E+000;
PDX1  				= +2.688E+000;
PDX2  				= -2.720E-001;
PDX3  				= +1.370E+001;
PEX1  				= +8.710E-001;
PEX2  				= -3.800E-002;
PEX3  				= +0.000E+000;
PEX4  				= +7.100E-002;
PKX1  				= +8.125E+001;
PKX2  				= -2.025E+001;
PKX3  				= +5.000E-001;
PHX1  				= +0.000E+000;
PHX2  				= +0.000E+000;
PVX1  				= +0.000E+000;
PVX2  				= +0.000E+000;
% =======================================================================
% RL
i = 0;
Fz = FZ_RL;
GAMMA = Sturzwinkel;
FX_RL = zeros((0.3/0.01+1),3);                                                % Vorinitialisierung
for KAPPA = 0:0.01:0.3
    % ====================================================================
    % Magic Formula Berechnung FX // Nur Längsschlupf
    GAMMA  =  GAMMA.*pi/180;
    FZ0PR  = FZ0  .*  LFZO;
    DFZ    = (Fz - FZ0PR) ./ FZ0PR;
    GAMMAX = GAMMA .* LGAX;
    SHX = (PHX1 + PHX2 .* DFZ) .* LHX;
    KAPPAX = KAPPA + SHX;
    CX = PCX1 .* LCX;
    MUX = (PDX1 + PDX2 .* DFZ) .* (1 - PDX3 .* GAMMAX.^2) .* LMUX;
    DX = MUX .* Fz;
    EX = (PEX1 + PEX2 .* DFZ + PEX3 .* DFZ.^2) .* (1 - PEX4 .* sign(KAPPAX)) .* LEX;
    KX = Fz .* (PKX1 + PKX2 .* DFZ) .* exp(PKX3 .* DFZ) .* LKX;
    BX = KX ./ (CX .* DX);
    SVX = Fz .* (PVX1 + PVX2 .* DFZ) .* LVX .* LMUX;
    % ====================================================================
    % Eintragung in die Matrix
    i=i+1;
    FX_RL(i,1) = Fz;
    FX_RL(i,2) = KAPPA;
    FX_RL(i,3) = DX .* sin(CX .* atan(BX .* KAPPAX - EX .* (BX .* KAPPAX - atan(BX .* KAPPAX)))) + SVX;
end
[~, Index] = max(FX_RL(:,3));                                               % Zeilennummer des maximalen FX-Werte
Schlupf_Ideal_RL = FX_RL(Index,2);                                          % Eintragung in die Ausgabegröße
% =======================================================================
% RR
i = 0;
Fz = FZ_RR;
GAMMA = Sturzwinkel;
FX_RR = zeros((0.3/0.01+1),3);                                                % Vorinitialisierung
for KAPPA = 0:0.01:0.3
    % ====================================================================
    % Magic Formula Berechnung FX // Nur Längsschlupf
    GAMMA  =  GAMMA.*pi/180;
    FZ0PR  = FZ0  .*  LFZO;
    DFZ    = (Fz - FZ0PR) ./ FZ0PR;
    GAMMAX = GAMMA .* LGAX;
    SHX = (PHX1 + PHX2 .* DFZ) .* LHX;
    KAPPAX = KAPPA + SHX;
    CX = PCX1 .* LCX;
    MUX = (PDX1 + PDX2 .* DFZ) .* (1 - PDX3 .* GAMMAX.^2) .* LMUX;
    DX = MUX .* Fz;
    EX = (PEX1 + PEX2 .* DFZ + PEX3 .* DFZ.^2) .* (1 - PEX4 .* sign(KAPPAX)) .* LEX;
    KX = Fz .* (PKX1 + PKX2 .* DFZ) .* exp(PKX3 .* DFZ) .* LKX;
    BX = KX ./ (CX .* DX);
    SVX = Fz .* (PVX1 + PVX2 .* DFZ) .* LVX .* LMUX;
    % ====================================================================
    % Eintragung in die Matrix
    i=i+1;
    FX_RR(i,1) = Fz;
    FX_RR(i,2) = KAPPA;
    FX_RR(i,3) = DX .* sin(CX .* atan(BX .* KAPPAX - EX .* (BX .* KAPPAX - atan(BX .* KAPPAX)))) + SVX;
end
[~, Index] = max(FX_RR(:,3));                                               % Zeilennummer des maximalen FX-Werte
Schlupf_Ideal_RR = FX_RR(Index,2);                                          % Eintragung in die Ausgabegröße

== matlab function Fahrdynamikregelung/Regelung/TUC/MATLAB Function ==
  data: SlipAngle_Ist_RL input; SlipAngle_Ist_RR input; SlipAngle_Ideal_RL input; SlipAngle_Ideal_RR input; SR_RL output; SR_RR output; Schlupf_Ist_RL input; Schlupf_Ist_RR input; Schlupf_Ideal_RL input; Schlupf_Ideal_RR input; Kappa_x_RL output; Kappa_x_RR output; Alpha_y_RL output; Alpha_y_RR output
function [SR_RL,SR_RR,Kappa_x_RL,Kappa_x_RR,Alpha_y_RL,Alpha_y_RR] = Schlupfausnutzung(SlipAngle_Ist_RL,SlipAngle_Ist_RR,SlipAngle_Ideal_RL,SlipAngle_Ideal_RR,...
    Schlupf_Ist_RL,Schlupf_Ist_RR,Schlupf_Ideal_RL,Schlupf_Ideal_RR)

    % Schlupfausnutzung RL
    Kappa_x_RL = Schlupf_Ist_RL/Schlupf_Ideal_RL;
    Alpha_y_RL = SlipAngle_Ist_RL/SlipAngle_Ideal_RL;
    SR_RL = sqrt(Kappa_x_RL^2 + Alpha_y_RL^2);

    % Schlupfausnutzung RR
    Kappa_x_RR = Schlupf_Ist_RR/Schlupf_Ideal_RR;
    Alpha_y_RR = SlipAngle_Ist_RR/SlipAngle_Ideal_RR;
    SR_RR = sqrt(Kappa_x_RR^2 + Alpha_y_RR^2);

== matlab function Fahrdynamikregelung/Regelung/TV/Verteilung Links//Rechts ==
  data: APPS input; SAS input; u input; APPS_L output; APPS_R output
function [APPS_L,APPS_R] = fcn(APPS,SAS,u)

if SAS >= 0                                 % Rechtskurve, Links höheres Drehmoment gefordert
    APPS_L = APPS/100 + u;
    APPS_R = APPS/100 - u;
else                                        % Linkskurve, Rechts höheres Drehmoment gefordert
    APPS_L = APPS/100 - u;
    APPS_R = APPS/100 + u;
end

== matlab function Fahrdynamikregelung/MATLAB Function ==
  data: P_RL input; n_RL output; P_RR input; M_RL input; M_RR input; v_x input; SAS input; a_y input; n_RR output; t_H_fzg parameter; Dyn_Reifenradius parameter
function [n_RL,n_RR] = fcn(P_RL,P_RR,M_RL,M_RR,v_x,SAS,a_y,t_H_fzg, Dyn_Reifenradius)

if  (M_RL > 10 || M_RR > 10)
    n_RL = P_RL/(2*pi*M_RL);
    n_RR = P_RR/(2*pi*M_RR);
else

    % Umrechung von v_x in n_x_RL und n_x_RR
    if SAS >= 0                                                                                 % Rechtskurve, Rechtes Rad ist Innen
        n_RL = (v_x * (v_x^2/a_y + t_H_fzg/2)) / ((v_x^2/a_y) * (2*pi*Dyn_Reifenradius));
        n_RR = (v_x * (v_x^2/a_y - t_H_fzg/2)) / ((v_x^2/a_y) * (2*pi*Dyn_Reifenradius));
    else                                                                                        % Linkskurve, Linkes Rad innen
        n_RL = (v_x * (v_x^2/a_y - t_H_fzg/2)) / ((v_x^2/a_y) * (2*pi*Dyn_Reifenradius));
        n_RR = (v_x * (v_x^2/a_y + t_H_fzg/2)) / ((v_x^2/a_y) * (2*pi*Dyn_Reifenradius));
    end
end

== matlab function Fahrdynamikregelung/Regelung/DTD/Schlupfregelung ==
  data: APPS_L input; APPS_L_SR output; APPS_R input; SR_RL input; SR_RR input; APPS_R_SR output
function [APPS_L_SR,APPS_R_SR] = fcn(APPS_L,APPS_R,SR_RL,SR_RR)

    % Saturation
    if SR_RL >= 1.9
        SR_RL = 1.9;
    end
    if SR_RR >= 1.9
        SR_RR = 1.9;
    end
    
    % Schlupfregelfaktor
    if SR_RL >= SR_RR
        APPS_L_SR = APPS_L * (2-SR_RL);
        APPS_R_SR = APPS_R * (2-SR_RL);
    else
        APPS_L_SR = APPS_L * (2-SR_RR);
        APPS_R_SR = APPS_R * (2-SR_RR);
    end

== matlab function Fahrdynamikregelung/Regelung/Fahrzustand/Geometrischer Lenkwinkel ==
  data: delta_V_geom output; v_x input; a_y input; t_H_fzg parameter; l_fzg parameter; delta_V_mess input; delta_V_mess output
function [delta_V_geom,delta_V_mess]  = LenkwinkelGeom(v_x,a_y, t_H_fzg, l_fzg,delta_V_mess)

    delta_V_geom = atand(l_fzg/((v_x*v_x/a_y)+(t_H_fzg/2)));

== matlab function Fahrdynamikregelung/Regelung/TV/Einspurmodell ==
  data: psi_dot_ref output; delta_V_mess input; v_x input; rutsch_zahl output; m_fzg parameter; l_fzg parameter; l_V_fzg parameter; l_H_fzg parameter; c_alpha_V parameter; c_alpha_H parameter
function [psi_dot_ref, rutsch_zahl]   = Einspurmodell(delta_V_mess, v_x, m_fzg, l_fzg, l_V_fzg, l_H_fzg, c_alpha_V, c_alpha_H)
%#codegen

% Charakteristische Geschwindigkeit zum Quadrat
square_v_ch = c_alpha_V * c_alpha_H * l_fzg / (m_fzg * ((c_alpha_H * l_H_fzg) - (c_alpha_V * l_V_fzg)));

% Soll Gierrate
%psi_dot_ref = v_x * delta_V / (l_fzg * (1 + (v_x^2 / square_v_ch)));
psi_dot_ref = v_x * delta_V_mess / l_fzg;

rutsch_zahl = v_x^2/square_v_ch;
end

== matlab function Fahrdynamikregelung/Regelung/TUC/Lateraler Load Transfer ==
  data: LT_Lat_Rear output; a_y input; m_Rear parameter; t_H_fzg parameter; h_COG parameter
function LT_Lat_Rear  = LT_Lateral(a_y,m_Rear, t_H_fzg, h_COG)

    LT_Lat_Rear = m_Rear*a_y*h_COG / t_H_fzg;

== matlab function Fahrdynamikregelung/Regelung/TUC/Longitudinaler Load Transfer ==
  data: LT_Long output; a_x input; m_Front parameter; m_Rear parameter; l_fzg parameter; h_COG parameter
function LT_Long  = LT_Long( a_x,m_Front, m_Rear, l_fzg, h_COG)

    LT_Long = (m_Front+m_Rear)*a_x*h_COG / l_fzg;

== matlab function Fahrdynamikregelung/Regelung/TUC/Schlupf Rear Ist ==
  data: v_x input; a_y input; SAS input; Schlupf_Ist_RL output; n_RL input; n_RR input; Schlupf_Ist_RR output; Dyn_Reifenradius parameter; t_H_fzg parameter; n_x_FL output; n_x_FR output; n_x output
function [Schlupf_Ist_RL,Schlupf_Ist_RR,n_x_FL,n_x_FR,n_x]   = Schlupf_Ist(v_x,a_y,SAS,n_RL,n_RR,Dyn_Reifenradius,t_H_fzg)

    % Referenzdrehzahl
    n_x = v_x / (2*pi*Dyn_Reifenradius);

    % Umrechung von v_x in n_x_RL und n_x_RR
    if SAS >= 0                                                                                 % Rechtskurve, Rechtes Rad ist Innen
        n_x_FL = (v_x * (v_x^2/a_y + t_H_fzg/2)) / ((v_x^2/a_y) * (2*pi*Dyn_Reifenradius));
        n_x_FR = (v_x * (v_x^2/a_y - t_H_fzg/2)) / ((v_x^2/a_y) * (2*pi*Dyn_Reifenradius));
    else                                                                                        % Linkskurve, Linkes Rad innen
        n_x_FL = (v_x * (v_x^2/a_y - t_H_fzg/2)) / ((v_x^2/a_y) * (2*pi*Dyn_Reifenradius));
        n_x_FR = (v_x * (v_x^2/a_y + t_H_fzg/2)) / ((v_x^2/a_y) * (2*pi*Dyn_Reifenradius));
    end
    
    Schlupf_Ist_RL = (n_RL-n_x_FL)/n_x_FL;
    Schlupf_Ist_RR = (n_RR-n_x_FR)/n_x_FR;

== matlab function Fahrdynamikregelung/Regelung/TUC/Reifennormalkraft Rear ==
  data: FZ_RL output; LT_Long input; LT_Lat_Rear input; F_Aero_Rear input; FZ_RR output; m_Rear parameter
function [FZ_RL,FZ_RR] = Reifennormalkraft(LT_Long,LT_Lat_Rear,F_Aero_Rear, m_Rear)

    FZ_RL = (m_Rear*9.81)/2 + LT_Long/4 + LT_Lat_Rear/2 + F_Aero_Rear/2;    % Rechtskurve // Masse links steigt
    FZ_RR = (m_Rear*9.81)/2 + LT_Long/4 - LT_Lat_Rear/2 + F_Aero_Rear/2;    % Linkskurve // Masse rechts steigt

== matlab function Fahrdynamikregelung/Regelung/TUC/Abtriebskräfte Rear ==
  data: v_x input; F_Aero_Rear output; c_DA parameter; aero_balance_rear parameter
function F_Aero_Rear   = Abriebskraft(v_x,c_DA, aero_balance_rear)

    F_Aero_Rear = 0.5 * 1.225 * c_DA * v_x * v_x * aero_balance_rear;
